simulink model "sim2"  (R2015a)
settings: Solver=ode45  StartTime=0.0  StopTime=10.0  RelTol=1e-3
settings Model: Creator=Manoj  LastModifiedBy=Manoj

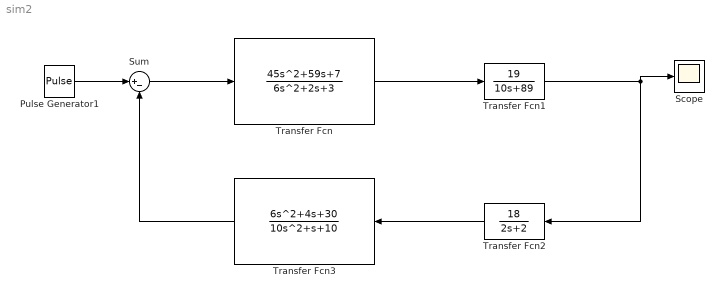
== system sim2 ==
  Pulse Generator1 : DiscretePulseGenerator  PulseType=Time based  Period=4  PhaseDelay=0-1
  Scope : Scope
      settings: TickLabels=on
  Sum : Sum  Inputs=|+-
  Transfer Fcn : TransferFcn  Numerator=[45 59 7]  Denominator=[6 2 3]
  Transfer Fcn1 : TransferFcn  Numerator=[19]  Denominator=[10 89]
  Transfer Fcn2 : TransferFcn  Numerator=[18]  Denominator=[2 2]
  Transfer Fcn3 : TransferFcn  Numerator=[6 4 30]  Denominator=[10 1 10]
  wires:
  Transfer Fcn/1 -> Transfer Fcn1/1
  Transfer Fcn2/1 -> Transfer Fcn3/1
  Transfer Fcn1/1 -> Transfer Fcn2/1, Scope/1
  Sum/1 -> Transfer Fcn/1
  Transfer Fcn3/1 -> Sum/2
  Pulse Generator1/1 -> Sum/1
